simulink model "Day6"  (R2023a)
settings: Solver=VariableStepAuto  StartTime=0.0  StopTime=10.0  RelTol=1e-3
undefined symbols (not defined in the file or in its folder): k
settings Model: Creator=Lenovo  LastModifiedBy=Lenovo

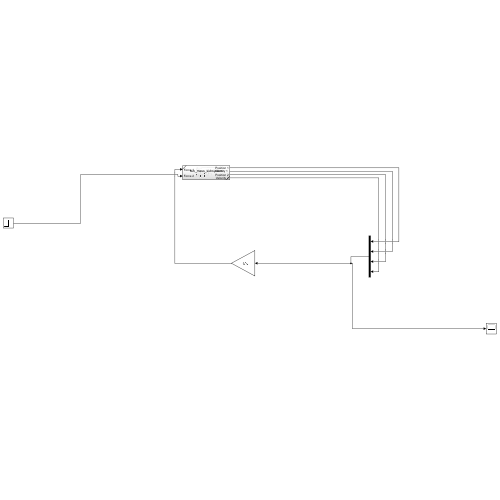
[thumbnail: Simulink's stored preview of the top-level diagram]
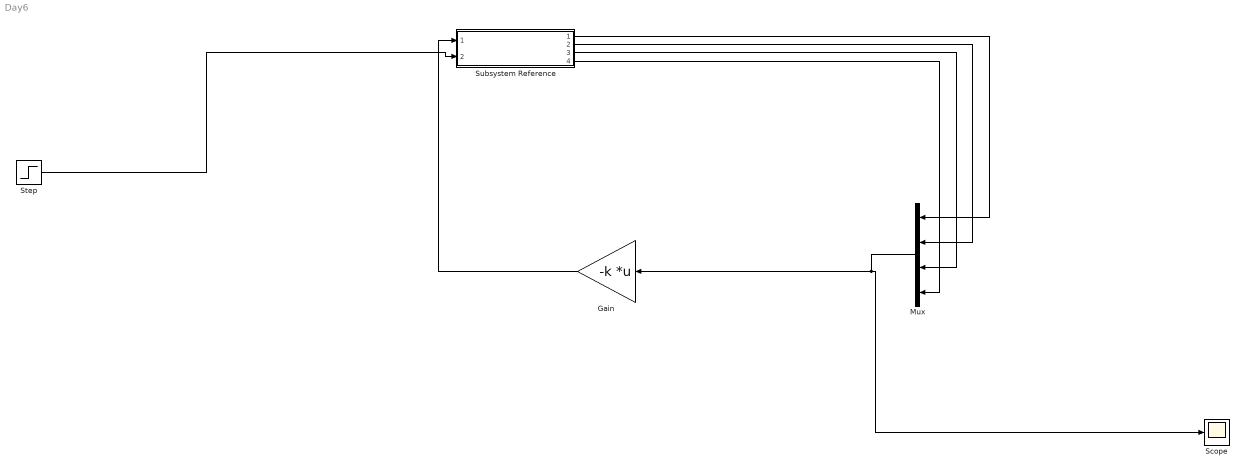
== system Day6 ==
  Gain : Gain  Gain=-k  Multiplication=Matrix(K*u)
  Mux : Mux
  Scope : Scope
  Step : Step  SampleTime=0
  Subsystem Reference : Subsystem  ReferencedSubsystem=two_mass_subsystem
  wires:
  Mux/1 -> Scope/1, Gain/1
  Subsystem Reference/1 -> Mux/1
  Subsystem Reference/2 -> Mux/2
  Subsystem Reference/3 -> Mux/3
  Subsystem Reference/4 -> Mux/4
  Step/1 -> Subsystem Reference/2
  Gain/1 -> Subsystem Reference/1
